simulink model "DiscTransController"  (Simulink 7.7)
settings: Solver=ode45  StartTime=0.0  StopTime=10.0  RelTol=1e-3
settings Model: Creator=jporter  LastModifiedBy=jporter

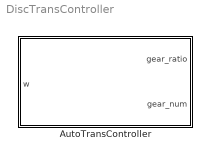
== system DiscTransController ==
  AutoTransController : Subsystem

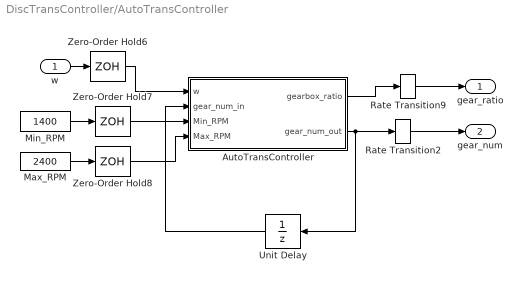
== system DiscTransController/AutoTransController ==
  w : Inport
  AutoTransController : Stateflow chart  TreatAsAtomicUnit=on
  Max_RPM : Constant  Value=2400
  Min_RPM : Constant  Value=1400
  Rate Transition2 : RateTransition  X0=1  OutPortSampleTime=0
  Rate Transition9 : RateTransition  X0=1  OutPortSampleTime=0
  Unit Delay : UnitDelay  SampleTime=-1
  Zero-Order Hold6 : ZeroOrderHold  Priority=-1  SampleTime=0.1
  Zero-Order Hold7 : ZeroOrderHold  Priority=-1  SampleTime=0.1
  Zero-Order Hold8 : ZeroOrderHold  Priority=-1  SampleTime=0.1
  gear_ratio : Outport
  gear_num : Outport  Port=2
  wires:
  AutoTransController/1(gearbox_ratio) -> Rate Transition9/1
  AutoTransController/2(gear_num_out) -> Unit Delay/1, Rate Transition2/1
  w/1 -> Zero-Order Hold6/1
  Unit Delay/1 -> AutoTransController/2(gear_num_in)
  Min_RPM/1 -> Zero-Order Hold7/1
  Max_RPM/1 -> Zero-Order Hold8/1
  Zero-Order Hold6/1 -> AutoTransController/1(w)
  Zero-Order Hold7/1 -> AutoTransController/3(Min_RPM)
  Zero-Order Hold8/1 -> AutoTransController/4(Max_RPM)
  Rate Transition9/1 -> gear_ratio/1
  Rate Transition2/1 -> gear_num/1

== matlab function AutoTransController/AutoTransController ==
  data: gearbox_ratio output double; w input double; gear_num_out output double; gear_num_in input double; Min_RPM input double; Max_RPM input double
function [gearbox_ratio, gear_num_out] = fcn(w, gear_num_in, Min_RPM, Max_RPM)
%#eml

%Min_RPM = 1400;
%Max_RPM = 2400;

gear_num_out = gear_num_in;
gearbox_ratio = 0.12/1;


if (w > (Max_RPM*2*pi/60)) && (gear_num_in < 4)
    gear_num_out = gear_num_in + 1;    
elseif (w < (Min_RPM*2*pi/60)) && (gear_num_in > 1)
    gear_num_out = gear_num_in - 1;
end

if (gear_num_in < 1)
    gear_num_out = 1;
end

if (gear_num_in > 4)
    gear_num_out = 4;
end

switch gear_num_out
    case 1
        gearbox_ratio = 0.12/3.5;
    case 2
        gearbox_ratio = 0.12/2.2;        
    case 3
        gearbox_ratio = 0.12/1.4;        
    case 4
        gearbox_ratio = 0.12/1;
end
